simulink model "simulink_sfunt_test_"  (R2022b)
settings: Solver=VariableStepAuto  StartTime=0.0  StopTime=10.0  RelTol=1e-3
settings Model: Creator=23776  LastModifiedBy=23776

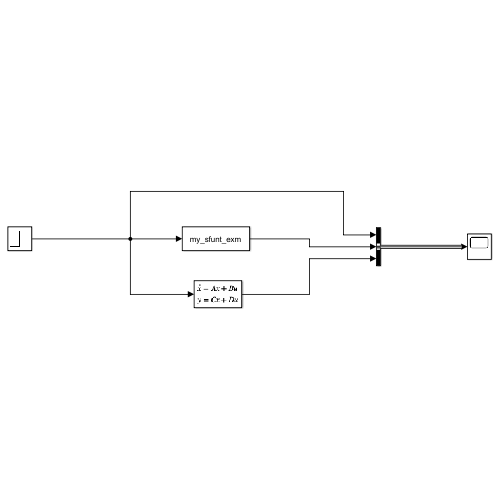
[thumbnail: Simulink's stored preview of the top-level diagram]
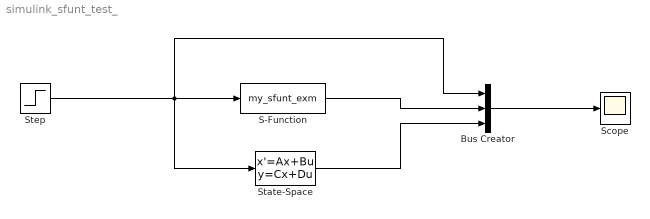
== system simulink_sfunt_test_ ==
  Bus Creator : BusCreator  Inputs=3
  S-Function : S-Function  FunctionName=my_sfunt_exm  SFunctionDeploymentMode=off  EnableBusSupport=off
  Scope : Scope
  State-Space : StateSpace  A=[ 0 1 ; -1/80 -3/10]  B=[ 0 ; 3/16 ]  C=[ 1 0 ]  D=0  InitialCondition=0
  Step : Step  SampleTime=0
  wires:
  Bus Creator/1 -> Scope/1
  Step/1 -> Bus Creator/1, State-Space/1, S-Function/1
  S-Function/1 -> Bus Creator/2
  State-Space/1 -> Bus Creator/3
